simulink model "BatMod_test"  (R2017a)
settings: Solver=VariableStepAuto  StartTime=0.0  StopTime=17  MaxStep=1e-3  RelTol=1e-3
libraries: simulink x1
settings Model: Creator=erich  LastModifiedBy=erich

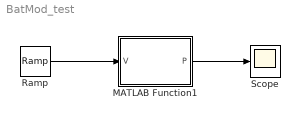
== system BatMod_test ==
  MATLAB Function1 : MATLAB Function  TreatAsAtomicUnit=on
  Ramp : simulink/Sources/Ramp  slope=1  start=0  X0=0
  Scope : Scope
  wires:
  MATLAB Function1/1(P) -> Scope/1
  Ramp/1 -> MATLAB Function1/1(V)

== matlab function BatMod_test/MATLAB Function1 ==
  data: V input; P output
function P = fcn(V)

P=0;
m=0;
b=0;

vfull = 16;
vexp = 14;
vnom = 8;

m1 = 11000/12;
m2 = 1000/(vexp-vnom);
m3 = 10*(1000/(vexp-vnom));

b1 = 0;
b2 = m1*vnom-m2*vnom;
b3 = m2*vexp+b2-m3*vexp;

if(V>=0 && V<vnom)
    m=m1;
    b=b1;
end

if(V>=vnom && V<vexp)
    m=m2;
    b=b2;
end

if(V>=vexp)
    m=m3;
    b=b3;
end

P=m*V + b;

if(V<0)
    P=0;
end
